simulink model "Pendulum_LP"  (R2024b)
settings: Solver=FixedStepAuto  StartTime=0.0  StopTime=30  FixedStep=0.001  RelTol=1e-3
values from neighbouring files (symbols this model uses):
  P1 = 0.7065    [main_LP.m]    (also in main_LP_w_regulator.m = -0.7065; main_LP_w_regulator_non_linear.m = -0.7065)
  P2 = 1.44    [main_LP.m]    (also in main_LP_w_regulator.m = -1.44; main_LP_w_regulator_non_linear.m = -1.44)
  P3 = 0.05622    [main_LP.m]    (also in main_LP_w_regulator.m; main_LP_w_regulator_non_linear.m)
  P4 = 0.008979    [main_LP.m]    (also in main_LP_w_regulator.m; main_LP_w_regulator_non_linear.m)
  P5 = 0.00232    [main_LP.m]    (also in main_LP_w_regulator.m; main_LP_w_regulator_non_linear.m)
  P6 = 1    [main_LP.m]    (also in main_LP_w_regulator.m; main_LP_w_regulator_non_linear.m)
  phi_dot_dot_sat = 100    [main_LP.m]    (also in main_LP_w_regulator.m; main_LP_w_regulator_non_linear.m)
  phi_dot_dot_threshold = 1e-10    [main_LP.m]    (also in main_LP_w_regulator.m; main_LP_w_regulator_non_linear.m)
  tau_a_sat = inf    [main_LP.m]    (also in main_LP_w_regulator.m; main_LP_w_regulator_non_linear.m)
  tau_a_threshold = 1e-10    [main_LP.m]    (also in main_LP_w_regulator.m; main_LP_w_regulator_non_linear.m)
  theta_dot_dot_sat = 100    [main_LP.m]    (also in main_LP_w_regulator.m; main_LP_w_regulator_non_linear.m)
  theta_dot_dot_threshold = 1e-10    [main_LP.m]    (also in main_LP_w_regulator.m; main_LP_w_regulator_non_linear.m)
settings Model: Creator=sipak  LastModifiedBy=sipak

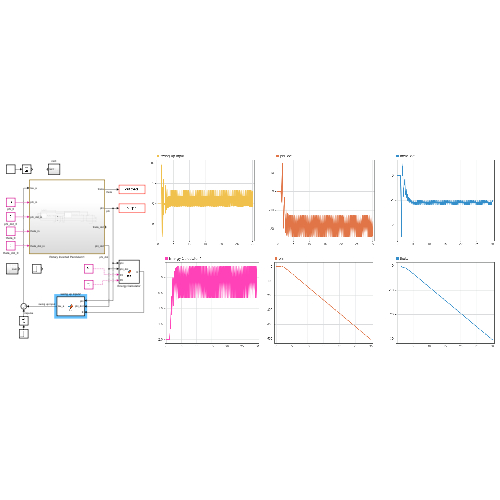
[thumbnail: Simulink's stored preview of the top-level diagram]
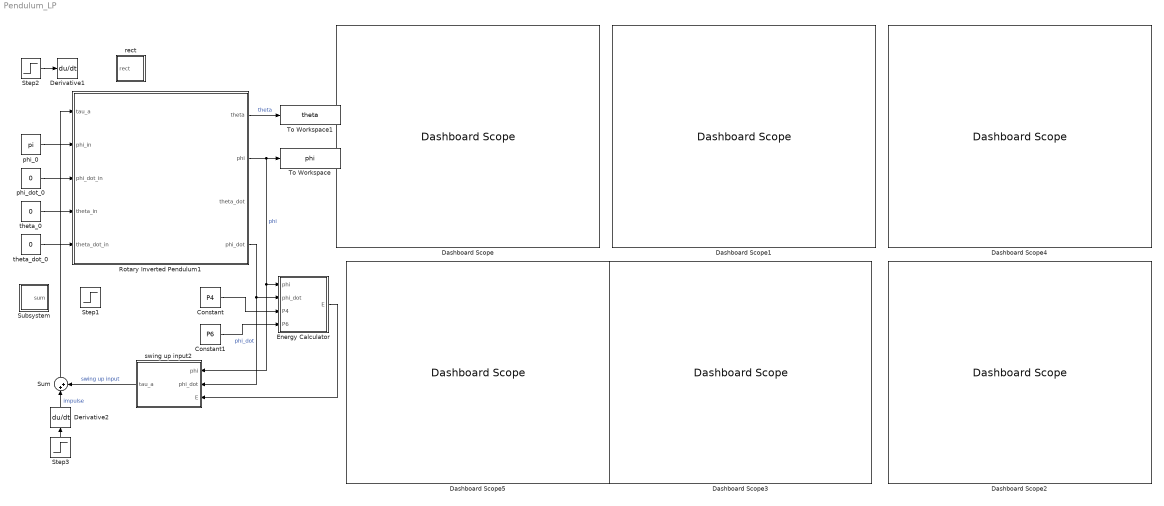
== system Pendulum_LP ==
  Constant : Constant  Value=P4
  Constant1 : Constant  Value=P6
  Dashboard Scope{,1..5} (6 alike) : DashboardScope
  Derivative1 : Derivative
  Derivative2 : Derivative
  Energy Calculator : MATLAB Function  TreatAsAtomicUnit=on
  Rotary Inverted Pendulum1 : Subsystem
  Step1 : Step  After=10  SampleTime=0
  Step2 : Step  After=1e10  SampleTime=0
  Step3 : Step  SampleTime=0
  Subsystem : Subsystem
  Sum : Sum  Inputs=|++
  To Workspace : ToWorkspace  VariableName=phi  SampleTime=-1
      settings: Save2DSignal=2-D array (concatenate along first dimension)
  To Workspace1 : ToWorkspace  VariableName=theta  SampleTime=-1
      settings: Save2DSignal=2-D array (concatenate along first dimension)
  phi_0 : Constant  Value=pi
  phi_dot_0 : Constant  Value=0
  rect : Subsystem
  swing up input2 : MATLAB Function  TreatAsAtomicUnit=on
  theta_0 : Constant  Value=0
  theta_dot_0 : Constant  Value=0
  wires:
  phi_dot_0/1 -> Rotary Inverted Pendulum1/3(phi_dot_in)
  phi_0/1 -> Rotary Inverted Pendulum1/2(phi_in)
  theta_dot_0/1 -> Rotary Inverted Pendulum1/5(theta_dot_in)
  Step2/1 -> Derivative1/1
  theta_0/1 -> Rotary Inverted Pendulum1/4(theta_in)
  Constant/1 -> Energy Calculator/3(P4)
  Constant1/1 -> Energy Calculator/4(P6)
  Rotary Inverted Pendulum1/2(phi) -> swing up input2/1(phi), Energy Calculator/1(phi), To Workspace/1  "phi"
  Rotary Inverted Pendulum1/1(theta) -> To Workspace1/1  "theta"
  Rotary Inverted Pendulum1/4(phi_dot) -> swing up input2/2(phi_dot), Energy Calculator/2(phi_dot)  "phi_dot"
  Energy Calculator/1(E) -> swing up input2/3(E)
  Step3/1 -> Derivative2/1
  swing up input2/1(tau_a) -> Sum/2  "swing up input"
  Derivative2/1 -> Sum/1  "impulse"
  Sum/1 -> Rotary Inverted Pendulum1/1(tau_a)

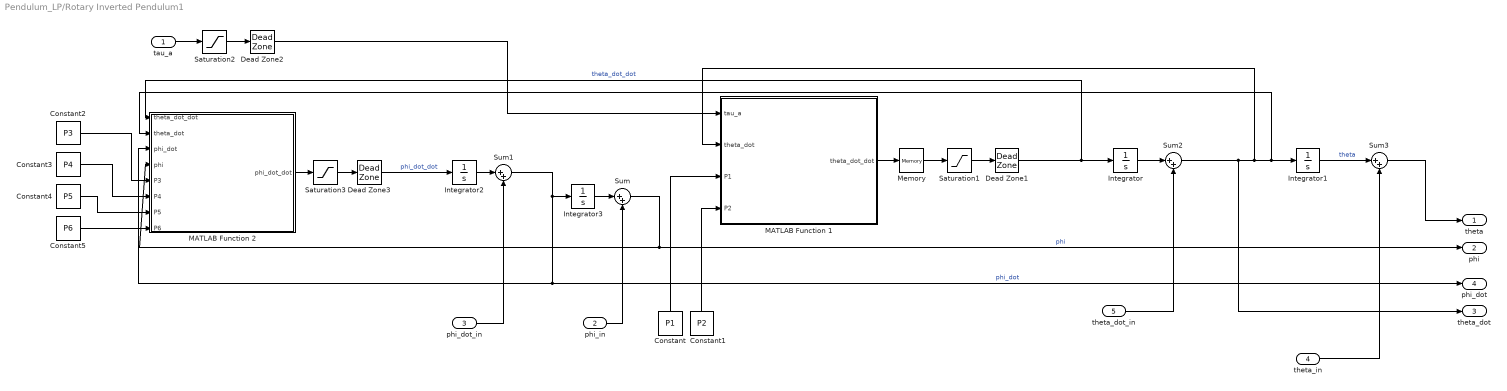
== system Pendulum_LP/Rotary Inverted Pendulum1 ==
  tau_a : Inport
  phi_in : Inport  Port=2
  phi_dot_in : Inport  Port=3
  theta_in : Inport  Port=4
  theta_dot_in : Inport  Port=5
  Constant : Constant  Value=P1
  Constant1 : Constant  Value=P2
  Constant2 : Constant  Value=P3
  Constant3 : Constant  Value=P4
  Constant4 : Constant  Value=P5
  Constant5 : Constant  Value=P6
  Dead Zone1 : DeadZone  LowerValue=-theta_dot_dot_threshold  UpperValue=theta_dot_dot_threshold
  Dead Zone2 : DeadZone  LowerValue=-tau_a_threshold  UpperValue=tau_a_threshold
  Dead Zone3 : DeadZone  LowerValue=-phi_dot_dot_threshold  UpperValue=phi_dot_dot_threshold
  Integrator{,1..3} (4 alike) : Integrator
  MATLAB Function 1 : MATLAB Function  TreatAsAtomicUnit=on
  MATLAB Function 2 : MATLAB Function  TreatAsAtomicUnit=on
  Memory : Memory
  Saturation1 : Saturate  UpperLimit=theta_dot_dot_sat  LowerLimit=-theta_dot_dot_sat
  Saturation2 : Saturate  UpperLimit=tau_a_sat  LowerLimit=-tau_a_sat
  Saturation3 : Saturate  UpperLimit=phi_dot_dot_sat  LowerLimit=-phi_dot_dot_sat
  Sum{,1..3} (4 alike) : Sum  Inputs=|++
  theta : Outport
  phi : Outport  Port=2
  theta_dot : Outport  Port=3
  phi_dot : Outport  Port=4
  wires:
  Integrator2/1 -> Sum1/1
  Integrator/1 -> Sum2/1
  Sum/1 -> phi/1, MATLAB Function 2/4(phi)  "phi"
  MATLAB Function 2/1(phi_dot_dot) -> Saturation3/1
  phi_in/1 -> Sum/2
  tau_a/1 -> Saturation2/1
  Integrator3/1 -> Sum/1
  theta_dot_in/1 -> Sum2/2
  phi_dot_in/1 -> Sum1/2
  MATLAB Function 1/1(theta_dot_dot) -> Memory/1
  Memory/1 -> Saturation1/1
  Sum1/1 -> phi_dot/1, MATLAB Function 2/3(phi_dot), Integrator3/1  "phi_dot"
  Sum2/1 -> MATLAB Function 1/2(theta_dot), MATLAB Function 2/2(theta_dot), Integrator1/1, theta_dot/1
  Saturation2/1 -> Dead Zone2/1
  Dead Zone2/1 -> MATLAB Function 1/1(tau_a)
  Dead Zone3/1 -> Integrator2/1  "phi_dot_dot"
  Saturation3/1 -> Dead Zone3/1
  Saturation1/1 -> Dead Zone1/1
  Dead Zone1/1 -> MATLAB Function 2/1(theta_dot_dot), Integrator/1  "theta_dot_dot"
  Constant2/1 -> MATLAB Function 2/5(P3)
  Constant4/1 -> MATLAB Function 2/7(P5)
  Constant3/1 -> MATLAB Function 2/6(P4)
  Constant5/1 -> MATLAB Function 2/8(P6)
  Constant/1 -> MATLAB Function 1/3(P1)
  Constant1/1 -> MATLAB Function 1/4(P2)
  theta_in/1 -> Sum3/2
  Integrator1/1 -> Sum3/1  "theta"
  Sum3/1 -> theta/1

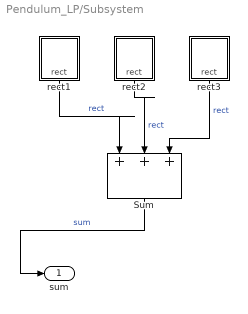
== system Pendulum_LP/Subsystem ==
  Sum : Sum  Inputs=|+++
  rect1 : Subsystem
  rect2 : Subsystem
  rect3 : Subsystem
  sum : Outport
  wires:
  Sum/1 -> sum/1  "sum"
  rect1/1(rect) -> Sum/1  "rect"
  rect2/1(rect) -> Sum/2  "rect"
  rect3/1(rect) -> Sum/3  "rect"

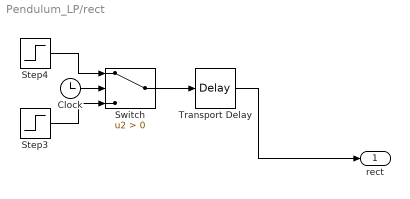
== system Pendulum_LP/rect ==
  Clock : Clock
  Step3 : Step  After=5  SampleTime=0
  Step4 : Step  Time=2  Before=5  After=0  SampleTime=0
  Switch : Switch  Criteria=u2 > Threshold  SaturateOnIntegerOverflow=off  InputSameDT=off
  Transport Delay : TransportDelay  DelayTime=0.3
  rect : Outport
  wires:
  Clock/1 -> Switch/2
  Step3/1 -> Switch/3
  Switch/1 -> Transport Delay/1
  Step4/1 -> Switch/1
  Transport Delay/1 -> rect/1

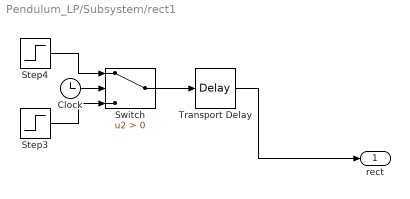
== system Pendulum_LP/Subsystem/rect1 ==
  Clock : Clock
  Step3 : Step  After=5  SampleTime=0
  Step4 : Step  Time=2  Before=5  After=0  SampleTime=0
  Switch : Switch  Criteria=u2 > Threshold  SaturateOnIntegerOverflow=off  InputSameDT=off
  Transport Delay : TransportDelay
  rect : Outport
  wires:
  Transport Delay/1 -> rect/1
  Step4/1 -> Switch/1
  Switch/1 -> Transport Delay/1
  Step3/1 -> Switch/3
  Clock/1 -> Switch/2

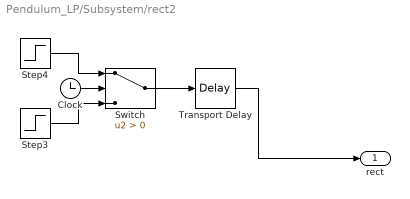
== system Pendulum_LP/Subsystem/rect2 ==
  Clock : Clock
  Step3 : Step  After=-5  SampleTime=0
  Step4 : Step  Time=2  Before=-5  After=0  SampleTime=0
  Switch : Switch  Criteria=u2 > Threshold  SaturateOnIntegerOverflow=off  InputSameDT=off
  Transport Delay : TransportDelay  DelayTime=4
  rect : Outport
  wires:
  Clock/1 -> Switch/2
  Step3/1 -> Switch/3
  Switch/1 -> Transport Delay/1
  Step4/1 -> Switch/1
  Transport Delay/1 -> rect/1

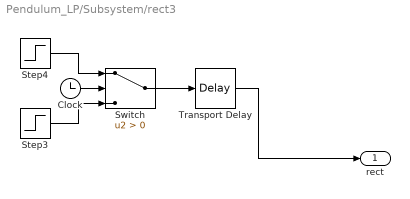
== system Pendulum_LP/Subsystem/rect3 ==
  Clock : Clock
  Step3 : Step  After=5  SampleTime=0
  Step4 : Step  Time=2  Before=5  After=0  SampleTime=0
  Switch : Switch  Criteria=u2 > Threshold  SaturateOnIntegerOverflow=off  InputSameDT=off
  Transport Delay : TransportDelay  DelayTime=7
  rect : Outport
  wires:
  Transport Delay/1 -> rect/1
  Step4/1 -> Switch/1
  Switch/1 -> Transport Delay/1
  Step3/1 -> Switch/3
  Clock/1 -> Switch/2

== matlab function Pendulum_LP/swing up input2 ==
  data: phi input; phi_dot input; E input; tau_a output
function tau_a = fcn(phi, phi_dot, E)
    k_swing = 5;
    E_target = 0;
    tau_a = k_swing * (E_target-E) * sign(phi_dot * cos(phi));

end

== matlab function Pendulum_LP/Energy Calculator ==
  data: phi input; phi_dot input; P4 input; E output; P6 input
function E = fcn(phi, phi_dot, P4, P6)
    % P4 = 2 * Ip_x2
    % P6 = mp * g * l

    omega0 = sqrt(P6 / (P4/2));
    E = P6 * (0.5 * (phi_dot / omega0)^2 + cos(phi) - 1);
    
end

== matlab function Pendulum_LP/Rotary Inverted Pendulum1/MATLAB Function 1 ==
  data: tau_a input; theta_dot_dot output; theta_dot input; P1 input; P2 input
function theta_dot_dot = equation1(tau_a, theta_dot, P1, P2)

    theta_dot_dot = (tau_a - (P2 * theta_dot)) / P1;
    
end

== matlab function Pendulum_LP/Rotary Inverted Pendulum1/MATLAB Function 2 ==
  data: theta_dot_dot input; phi_dot_dot output; theta_dot input; phi_dot input; phi input; P3 input; P4 input; P5 input; P6 input
function phi_dot_dot = equation2(theta_dot_dot, theta_dot, phi_dot, phi, P3, P4, P5, P6)

    tau_p = 0;
    phi_dot_dot = (2 * tau_p - (P3 * theta_dot_dot * cos(phi)) ...
                   + (0 * theta_dot^2 * sin(2 * phi)) ... % We put 0 times the rest because Ip_y2 disappear when linearizing. That might be false
                   + (P6 * sin(phi)) ...
                   - (P5 * phi_dot)) / P4;
end
